simulink model "pendulumWithoutDamping"  (Simulink 7.2)
settings: Solver=ode45  StartTime=0.0  StopTime=10.0  RelTol=1e-3
undefined symbols (not defined in the file or in its folder): g, L
libraries: simulink x1
settings Model: Creator=mauricio  LastModifiedBy=mauricio

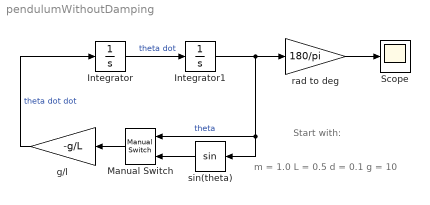
== system pendulumWithoutDamping ==
  note: Start with:
  note: m = 1.0
      | L = 0.5
      |  d = 0.1
      | g = 10
  Integrator : Integrator
  Integrator1 : Integrator  InitialCondition=pi/6
  Manual Switch : simulink/Signal Routing/Manual Switch  Orientation=left  SystemSampleTime=-1  sw=0  action=0  varsize=off
  Scope : Scope
      settings: YMin=-45  YMax=45
  g/l : Gain  Orientation=left  Gain=-g/L  ParameterDataType=sfix(16)  ParameterScaling=2^0  OutDataType=sfix(16)  OutScaling=2^0
  rad to deg : Gain  Gain=180/pi  ParameterDataType=sfix(16)  ParameterScaling=2^0  OutDataType=sfix(16)  OutScaling=2^0
  sin(theta) : Trigonometry  Orientation=left
  wires:
  Integrator/1 -> Integrator1/1  "theta dot"
  Integrator1/1 -> rad to deg/1, sin(theta)/1, Manual Switch/1  "theta"
  g/l/1 -> Integrator/1  "theta dot dot"
  rad to deg/1 -> Scope/1
  sin(theta)/1 -> Manual Switch/2
  Manual Switch/1 -> g/l/1
